simulink model "RCfilterslx"  (R2024a)
settings: Solver=FixedStepAuto  StartTime=0.0  StopTime=2  FixedStep=1e-6  RelTol=1e-3
libraries: mcbcontrolslib x1
settings Model: Creator=wsl  LastModifiedBy=wsl

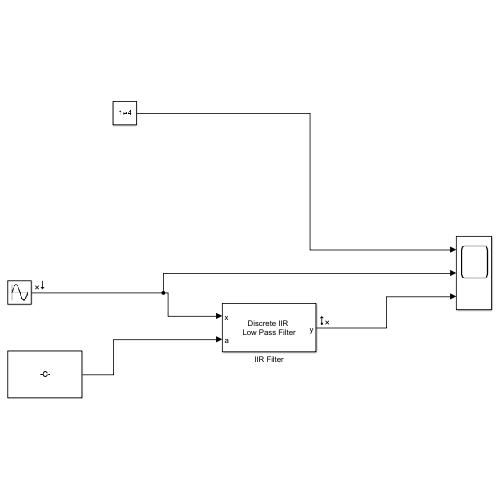
[thumbnail: Simulink's stored preview of the top-level diagram]
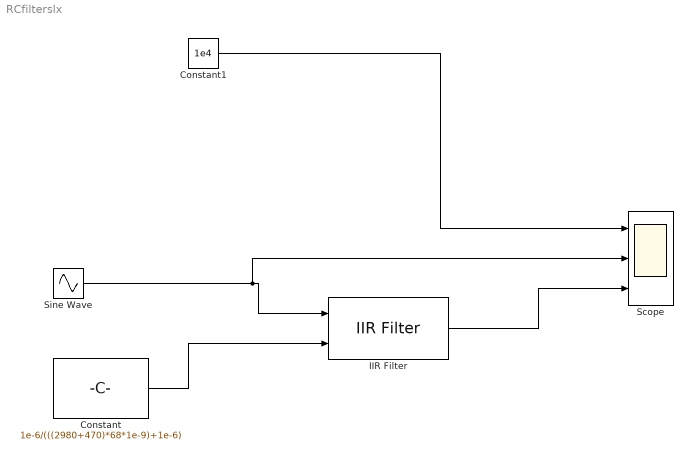
== system RCfilterslx ==
  Constant : Constant  Value=1e-6/(((2980+470)*68*1e-9)+1e-6)
  Constant1 : Constant  Value=1e4
  IIR Filter : mcbcontrolslib/IIR Filter  VariantControl=Low Pass Filter  VariantSelect=Low-pass  FilterConstantInputType=Input port  Filter_constant=0.01  advancedSettings=off  Ts=50e-6  cutOff_freq=32.1525
      settings: LibrarySourceBlock=mcblib/Signal Management/IIR Filter
  Scope : Scope  NumInputPorts=3
  Sine Wave : Sin  Frequency=2*pi*670  SampleTime=0
  wires:
  Constant/1 -> IIR Filter/2
  Sine Wave/1 -> Scope/2, IIR Filter/1
  IIR Filter/1 -> Scope/3
  Constant1/1 -> Scope/1
